simulink model "SimPowACM601"  (R2018b)
settings: Solver=FixedStepAuto  StartTime=0.0  StopTime=Tmu*100  FixedStep=T0  MaxStep=T0  RelTol=1e-3
values from neighbouring files (symbols this model uses):
  add_error = 0    [MathACM601.m]
  ce = 0.0712    [MathACM601.m]
  Cf = 100e-6    (= 0.0001)    [MathACM601.m]
  cm = 0.0712    [MathACM601.m]
  dia = 0.002*Isc*kdt    (= 13.339872)    [MathACM601.m]
  dib = 0.003*Isc*kdt    (= 20.009808)    [MathACM601.m]
  dic = -0.009*Isc*kdt    (= -60.029424)    [MathACM601.m]
  Isc = Udc/R    (= 10.6666666667)    [MathACM601.m]
  J = 0.11e-4    (= 1.1e-05)    [MathACM601.m]
  k = 2    [MathACM601.m]
  KADC = (2^12-1)/3.3    (= 1240.90909091)    [MathACM601.m]
  kda = 1    [MathACM601.m]
  kdb = 0.99    [MathACM601.m]
  kdc = 1.015    [MathACM601.m]
  kdt = Rshunt*Kopa*KADC    (= 625.3065)    [MathACM601.m]
  Ki1 = 1/(Kob*Tt)    (= 375)    [MathACM601.m]
  Ki2 = J*2/(3*8*Tmu^2*ce)    (= 0.514981273408)    [MathACM601.m]
  Kopa = 1.527    [MathACM601.m]
  Kp1 = Te*Ki1    (= 0.5625)    [MathACM601.m]
  Kp2 = 4*Tmu*Ki2    (= 0.0102996254682)    [MathACM601.m]
  Kshunt = 0.001    [MathACM601.m]
  Kv = 1    [MathACM601.m]
  Lsa = Ls    (= 0.002)    [MathACM601.m]
  Lsb = Ls    (= 0.002)    [MathACM601.m]
  Lsc = Ls    (= 0.002)    [MathACM601.m]
  PreMod_3 = 0    [MathACM601.m]
  R = 0.75    [MathACM601.m]
  Ra = R    (= 0.75)    [MathACM601.m]
  Rb = R    (= 0.75)    [MathACM601.m]
  Rc = R    (= 0.75)    [MathACM601.m]
  Rshunt = 0.33    [MathACM601.m]
  Sw = 0    [MathACM601.m]
  T0 = 1e-6    (= 1e-06)    [MathACM601.m]
  tau = 0.00    (= 0)    [MathACM601.m]
  Te = R*Ls    (= 0.0015)    [MathACM601.m]
  Tpwm = 0.5e-4    (= 5e-05)    [MathACM601.m]
  Ts1 = 0.5e-4    (= 5e-05)    [MathACM601.m]
  Ts2 = 0.5e-3    (= 0.0005)    [MathACM601.m]
  Ubias = 1.558    [MathACM601.m]
  Udc = 8    [MathACM601.m]
  zp = 4    [MathACM601.m]
libraries: powerlib x23
settings Model: Creator=ivshu  LastModifiedBy=Шустов Илья
settings SFSimCC: SimUseLocalCustomCode=off
settings RTWCC: RTWUseLocalCustomCode=off
settings CodeAppCC: StateflowObjectComments=on
settings SimscapeCC: SimscapeNormalizeSystem=off

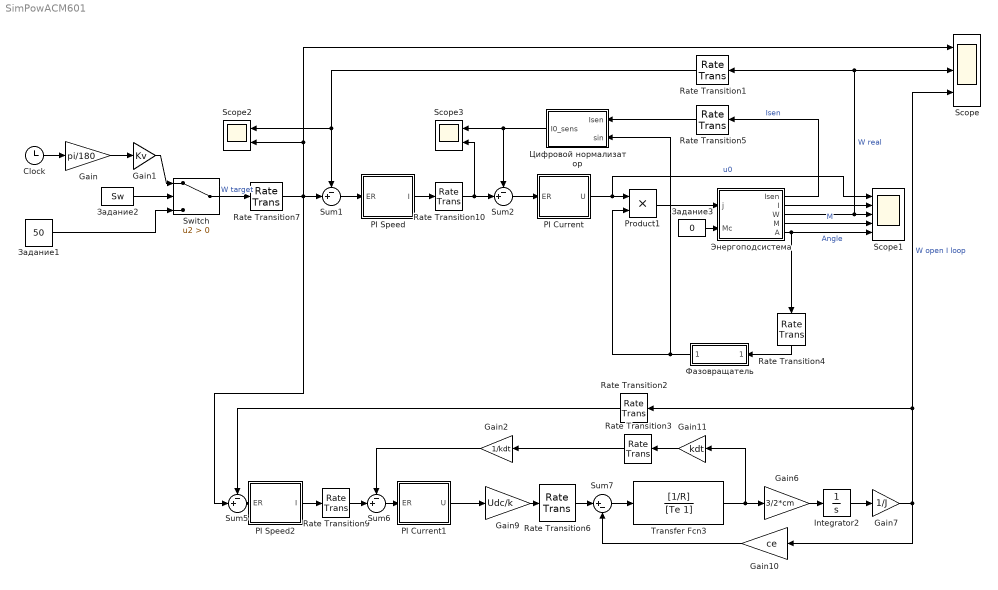
== system SimPowACM601 ==
  Clock : Clock
  Gain : Gain  Gain=pi/180
  Gain1 : Gain  Gain=Kv
  Gain10 : Gain  Gain=ce
  Gain11 : Gain  Gain=kdt
  Gain2 : Gain  Gain=1/kdt
  Gain6 : Gain  Gain=3/2*cm
  Gain7 : Gain  Gain=1/J
  Gain9 : Gain  Gain=Udc/k
  Integrator2 : Integrator
  PI Current : Subsystem
  PI Current1 : Subsystem
  PI Speed : Subsystem
  PI Speed2 : Subsystem
  Product1 : Product
  Rate Transition1 : RateTransition  OutPortSampleTime=Ts2
  Rate Transition{3..5,9..10} (5 alike) : RateTransition  OutPortSampleTime=Ts1
  Rate Transition2 : RateTransition  OutPortSampleTime=Ts2
  Rate Transition6 : RateTransition  OutPortSampleTimeOpt=Inherit
  Rate Transition7 : RateTransition  OutPortSampleTime=Ts2
  Scope : Scope  NumInputPorts=3
  Scope1 : Scope  NumInputPorts=5
  Scope2 : Scope  NumInputPorts=2
  Scope3 : Scope  NumInputPorts=2
  Sum{1..2,5..6} (4 alike) : Sum  Inputs=-+|
  Sum7 : Sum  Inputs=|+-
  Switch : Switch  Criteria=u2 > Threshold
  Transfer Fcn3 : TransferFcn  Numerator=[1/R]  Denominator=[Te 1]
  Задание1 : Constant  Value=50
  Задание2 : Constant  Value=Sw
  Задание3 : Constant  Value=0
  Фазовращатель : Subsystem
  Цифровой нормализатор : Subsystem
  Энергоподсистема : Subsystem
  wires:
  Product1/1 -> Энергоподсистема/1(j)
  Энергоподсистема/3(W) -> Scope1/3, Rate Transition1/1, Scope/2  "W real"
  Sum2/1 -> PI Current/1(ER)
  Цифровой нормализатор/1(I0_sens) -> Sum2/1, Scope3/1
  Rate Transition1/1 -> Sum1/1, Scope2/1
  Задание1/1 -> Switch/3
  Gain/1 -> Gain1/1
  Clock/1 -> Gain/1
  Gain1/1 -> Switch/1
  Энергоподсистема/5(A) -> Rate Transition4/1, Scope1/5  "Angle"
  Энергоподсистема/1(Isen) -> Rate Transition5/1  "Isen"
  Switch/1 -> Rate Transition7/1  "W target"
  Задание2/1 -> Switch/2
  Sum1/1 -> PI Speed/1(ER)
  Sum5/1 -> PI Speed2/1(ER)
  PI Speed2/1(I) -> Rate Transition9/1
  Sum6/1 -> PI Current1/1(ER)
  Transfer Fcn3/1 -> Gain6/1, Gain11/1
  Integrator2/1 -> Gain7/1
  Gain6/1 -> Integrator2/1
  Gain7/1 -> Gain10/1, Rate Transition2/1, Scope/3  "W open I loop"
  Rate Transition2/1 -> Sum5/1
  Rate Transition3/1 -> Gain2/1
  Sum7/1 -> Transfer Fcn3/1
  Rate Transition6/1 -> Sum7/1
  Gain10/1 -> Sum7/2
  Gain11/1 -> Rate Transition3/1
  PI Current/1(U) -> Scope1/1, Product1/1  "u0"
  Rate Transition7/1 -> Sum5/2, Sum1/2, Scope/1, Scope2/2
  Энергоподсистема/4(M) -> Scope1/4  "M"
  Фазовращатель/1(sin(3f)) -> Product1/2, Цифровой нормализатор/2(sin)
  Rate Transition4/1 -> Фазовращатель/1(Angle)
  Rate Transition5/1 -> Цифровой нормализатор/1(Isen)
  Gain9/1 -> Rate Transition6/1
  PI Current1/1(U) -> Gain9/1
  Задание3/1 -> Энергоподсистема/2(Mc)
  Gain2/1 -> Sum6/1
  PI Speed/1(I) -> Rate Transition10/1
  Энергоподсистема/2(I) -> Scope1/2
  Rate Transition9/1 -> Sum6/2
  Rate Transition10/1 -> Scope3/2, Sum2/2

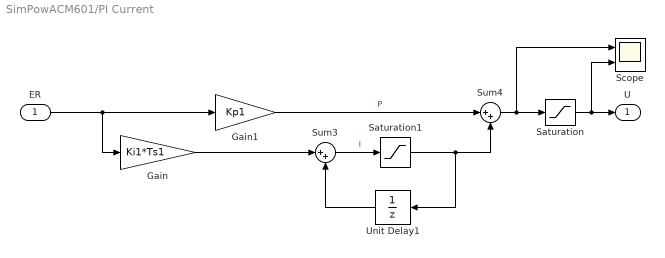
== system SimPowACM601/PI Current ==
  ER : Inport
  Gain : Gain  Gain=Ki1*Ts1
  Gain1 : Gain  Gain=Kp1
  Saturation : Saturate  UpperLimit=1  LowerLimit=-1
  Saturation1 : Saturate  UpperLimit=1  LowerLimit=-1
  Scope : Scope  NumInputPorts=2
  Sum3 : Sum  Inputs=|++
  Sum4 : Sum  Inputs=|++
  Unit Delay1 : UnitDelay  SampleTime=Ts1
  U : Outport
  wires:
  Saturation/1 -> Scope/2, U/1
  Sum4/1 -> Scope/1, Saturation/1
  Gain/1 -> Sum3/1
  Unit Delay1/1 -> Sum3/2
  Sum3/1 -> Saturation1/1  "I"
  Gain1/1 -> Sum4/1  "P"
  ER/1 -> Gain/1, Gain1/1
  Saturation1/1 -> Sum4/2, Unit Delay1/1

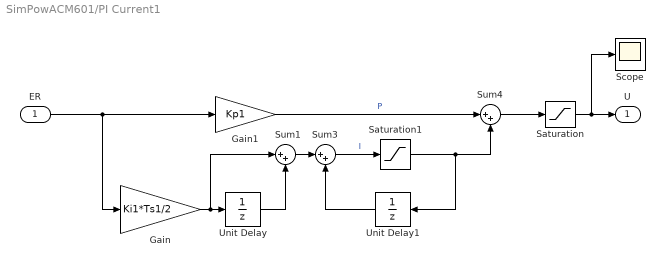
== system SimPowACM601/PI Current1 ==
  ER : Inport
  Gain : Gain  Gain=Ki1*Ts1/2
  Gain1 : Gain  Gain=Kp1
  Saturation : Saturate  UpperLimit=1  LowerLimit=-1
  Saturation1 : Saturate  UpperLimit=1  LowerLimit=-1
  Scope : Scope
  Sum1 : Sum  Inputs=|++
  Sum3 : Sum  Inputs=|++
  Sum4 : Sum  Inputs=|++
  Unit Delay : UnitDelay  SampleTime=Ts1
  Unit Delay1 : UnitDelay  SampleTime=Ts1
  U : Outport
  wires:
  Saturation/1 -> Scope/1, U/1
  Sum4/1 -> Saturation/1
  Gain/1 -> Sum1/1, Unit Delay/1
  Unit Delay/1 -> Sum1/2
  Sum1/1 -> Sum3/1
  Unit Delay1/1 -> Sum3/2
  Sum3/1 -> Saturation1/1  "I"
  Gain1/1 -> Sum4/1  "P"
  ER/1 -> Gain/1, Gain1/1
  Saturation1/1 -> Sum4/2, Unit Delay1/1

== system SimPowACM601/PI Speed ==
  ER : Inport
  Gain : Gain  Gain=Ki2*Ts2
  Gain1 : Gain  Gain=Kp2
  Saturation : Saturate  UpperLimit=Isc  LowerLimit=-Isc
  Saturation1 : Saturate  UpperLimit=Isc  LowerLimit=-Isc
  Scope : Scope  NumInputPorts=2
  Sum3 : Sum  Inputs=|++
  Sum4 : Sum  Inputs=|++
  Unit Delay1 : UnitDelay  SampleTime=Ts2
  I : Outport
  wires:
  Sum4/1 -> Saturation/1
  Gain/1 -> Sum3/1
  Unit Delay1/1 -> Sum3/2
  Sum3/1 -> Saturation1/1  "I"
  Gain1/1 -> Sum4/1  "P"
  ER/1 -> Gain/1, Gain1/1
  Saturation1/1 -> Scope/1, Sum4/2, Unit Delay1/1
  Saturation/1 -> Scope/2, I/1

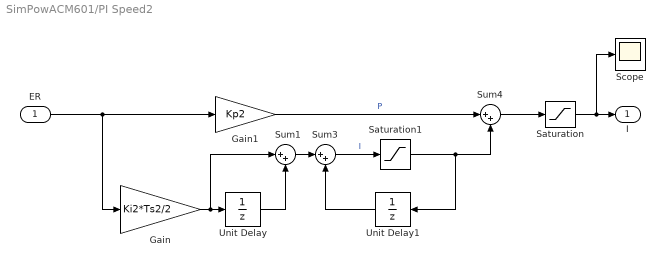
== system SimPowACM601/PI Speed2 ==
  ER : Inport
  Gain : Gain  Gain=Ki2*Ts2/2
  Gain1 : Gain  Gain=Kp2
  Saturation : Saturate  UpperLimit=Isc  LowerLimit=-Isc
  Saturation1 : Saturate  UpperLimit=Isc  LowerLimit=-Isc
  Scope : Scope
  Sum1 : Sum  Inputs=|++
  Sum3 : Sum  Inputs=|++
  Sum4 : Sum  Inputs=|++
  Unit Delay : UnitDelay  SampleTime=Ts2
  Unit Delay1 : UnitDelay  SampleTime=Ts2
  I : Outport
  wires:
  Sum4/1 -> Saturation/1
  Gain/1 -> Sum1/1, Unit Delay/1
  Unit Delay/1 -> Sum1/2
  Sum1/1 -> Sum3/1
  Unit Delay1/1 -> Sum3/2
  Sum3/1 -> Saturation1/1  "I"
  Gain1/1 -> Sum4/1  "P"
  ER/1 -> Gain/1, Gain1/1
  Saturation1/1 -> Sum4/2, Unit Delay1/1
  Saturation/1 -> Scope/1, I/1

== system SimPowACM601/Фазовращатель ==
  Angle : Inport
  Fcn1 : Fcn  Expr=sin(u(1))
  Fcn2 : Fcn  Expr=sin(u(1)+2*pi/3)
  Fcn3 : Fcn  Expr=sin(u(1)-2*pi/3)
  Gain2 : Gain  Gain=zp
  Mux2 : Mux  Inputs=3
  sin(3f) : Outport
  wires:
  Fcn2/1 -> Mux2/2
  Fcn3/1 -> Mux2/3
  Fcn1/1 -> Mux2/1
  Angle/1 -> Gain2/1
  Gain2/1 -> Fcn1/1, Fcn3/1, Fcn2/1
  Mux2/1 -> sin(3f)/1

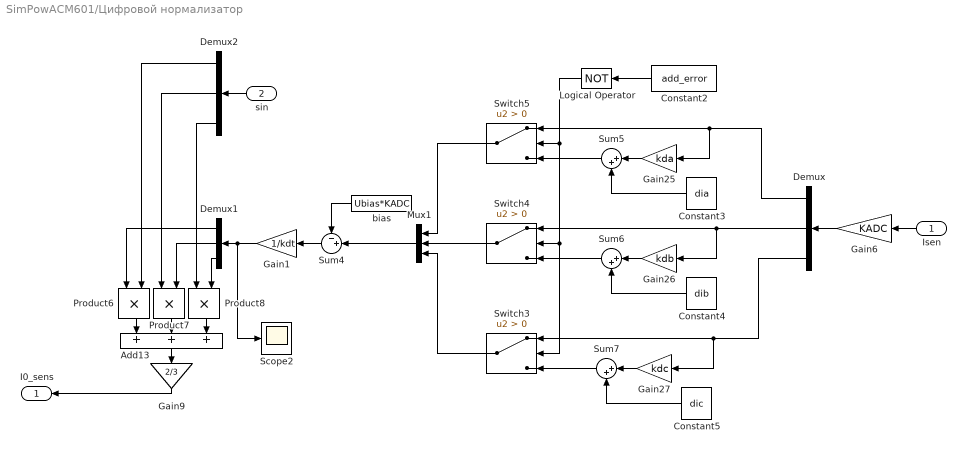
== system SimPowACM601/Цифровой нормализатор ==
  Isen : Inport
  sin : Inport  Port=2
  Add13 : Sum  Inputs=+++
  Constant2 : Constant  Value=add_error
  Constant3 : Constant  Value=dia
  Constant4 : Constant  Value=dib
  Constant5 : Constant  Value=dic
  Demux : Demux  Outputs=3
  Demux1 : Demux  Outputs=3
  Demux2 : Demux  Outputs=3
  Gain1 : Gain  Gain=1/kdt
  Gain25 : Gain  Gain=kda
  Gain26 : Gain  Gain=kdb
  Gain27 : Gain  Gain=kdc
  Gain6 : Gain  Gain=KADC
  Gain9 : Gain  Gain=2/3
  Logical Operator : Logic  Operator=NOT  AllPortsSameDT=off  OutDataTypeStr=boolean
  Mux1 : Mux  Inputs=3
  Product6 : Product
  Product7 : Product
  Product8 : Product
  Scope2 : Scope
  Sum4 : Sum  Inputs=-+|
  Sum5 : Sum  Inputs=|++
  Sum6 : Sum  Inputs=|++
  Sum7 : Sum  Inputs=|++
  Switch3 : Switch  Criteria=u2 > Threshold
  Switch4 : Switch  Criteria=u2 > Threshold
  Switch5 : Switch  Criteria=u2 > Threshold
  bias : Constant  Value=Ubias*KADC
  I0_sens : Outport
  wires:
  Switch4/1 -> Mux1/2
  Switch3/1 -> Mux1/3
  Switch5/1 -> Mux1/1
  Sum5/1 -> Switch5/3
  Constant2/1 -> Logical Operator/1
  Constant3/1 -> Sum5/2
  Gain25/1 -> Sum5/1
  Gain26/1 -> Sum6/1
  Isen/1 -> Gain6/1
  Sum6/1 -> Switch4/3
  Gain27/1 -> Sum7/1
  Sum7/1 -> Switch3/3
  Constant4/1 -> Sum6/2
  Constant5/1 -> Sum7/2
  Logical Operator/1 -> Switch4/2, Switch3/2, Switch5/2
  Demux/3 -> Gain27/1, Switch3/1
  Demux/2 -> Gain26/1, Switch4/1
  Demux/1 -> Gain25/1, Switch5/1
  bias/1 -> Sum4/1
  Sum4/1 -> Gain1/1
  Demux2/3 -> Product8/1
  Demux2/1 -> Product6/2
  Demux1/2 -> Product7/2
  Product6/1 -> Add13/1
  Product7/1 -> Add13/2
  Demux1/1 -> Product6/1
  Product8/1 -> Add13/3
  Gain9/1 -> I0_sens/1
  Add13/1 -> Gain9/1
  Demux1/3 -> Product8/2
  Mux1/1 -> Sum4/2
  Demux2/2 -> Product7/1
  sin/1 -> Demux2/1
  Gain6/1 -> Demux/1
  Gain1/1 -> Scope2/1, Demux1/1

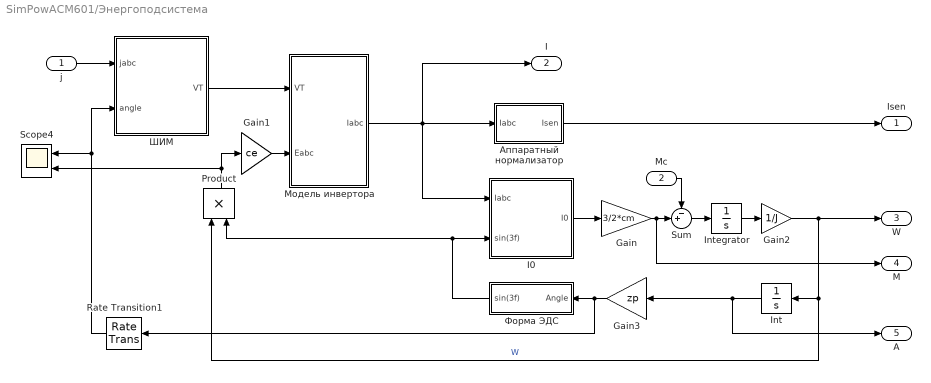
== system SimPowACM601/Энергоподсистема ==
  j : Inport
  Mc : Inport  Port=2
  Gain : Gain  Gain=3/2*cm
  Gain1 : Gain  Gain=ce
  Gain2 : Gain  Gain=1/J
  Gain3 : Gain  Gain=zp
  I0 : Subsystem
  Int : Integrator
  Integrator : Integrator
  Product : Product
  Rate Transition1 : RateTransition  OutPortSampleTime=Ts1
  Scope4 : Scope  NumInputPorts=2
  Sum : Sum  Inputs=-+|
  Аппаратный нормализатор : Subsystem
  Модель инвертора : Subsystem
  Форма ЭДС : Subsystem
  ШИМ : Subsystem
  Isen : Outport
  I : Outport  Port=2
  W : Outport  Port=3
  M : Outport  Port=4
  A : Outport  Port=5
  wires:
  Integrator/1 -> Gain2/1
  Gain2/1 -> Product/1, Int/1, W/1  "W"
  I0/1(I0) -> Gain/1
  Форма ЭДС/1(sin(3f)) -> Product/2, I0/2(sin(3f))
  Sum/1 -> Integrator/1
  Product/1 -> Gain1/1, Scope4/2
  Gain/1 -> M/1, Sum/2
  Модель инвертора/1(Iabc) -> I/1, Аппаратный нормализатор/1(Iabc), I0/1(Iabc)
  Mc/1 -> Sum/1
  Аппаратный нормализатор/1(Isen) -> Isen/1
  Int/1 -> A/1, Gain3/1
  ШИМ/1(VT) -> Модель инвертора/1(" VT")
  j/1 -> ШИМ/1(jabc)
  Gain3/1 -> Rate Transition1/1, Форма ЭДС/1(Angle)
  Gain1/1 -> Модель инвертора/2(" Eabc")
  Rate Transition1/1 -> ШИМ/2(angle), Scope4/1

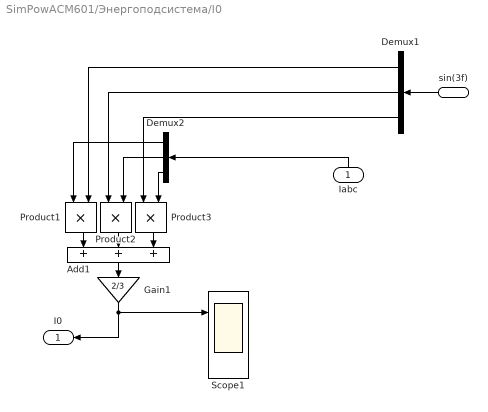
== system SimPowACM601/Энергоподсистема/I0 ==
  Iabc : Inport
  sin(3f) : Inport  Port=2
  Add1 : Sum  Inputs=+++
  Demux1 : Demux  Outputs=3
  Demux2 : Demux  Outputs=3
  Gain1 : Gain  Gain=2/3
  Product1 : Product
  Product2 : Product
  Product3 : Product
  Scope1 : Scope  NumInputPorts=2
  I0 : Outport
  wires:
  sin(3f)/1 -> Demux1/1
  Demux1/3 -> Product3/1
  Demux1/2 -> Product2/1
  Demux1/1 -> Product1/2
  Product3/1 -> Add1/3
  Demux2/1 -> Product1/1
  Add1/1 -> Gain1/1
  Demux2/3 -> Product3/2
  Iabc/1 -> Demux2/1
  Product1/1 -> Add1/1
  Product2/1 -> Add1/2
  Demux2/2 -> Product2/2
  Gain1/1 -> Scope1/1, I0/1

== system SimPowACM601/Энергоподсистема/Аппаратный нормализатор ==
  Iabc : Inport
  Constant1 : Constant  Value=Ubias
  Gain1 : Gain  Gain=Rshunt
  Gain30 : Gain  Gain=Kopa
  Sum1 : Sum  Inputs=++|
  Isen : Outport
  wires:
  Iabc/1 -> Gain1/1
  Constant1/1 -> Sum1/1
  Gain30/1 -> Sum1/2
  Sum1/1 -> Isen/1
  Gain1/1 -> Gain30/1

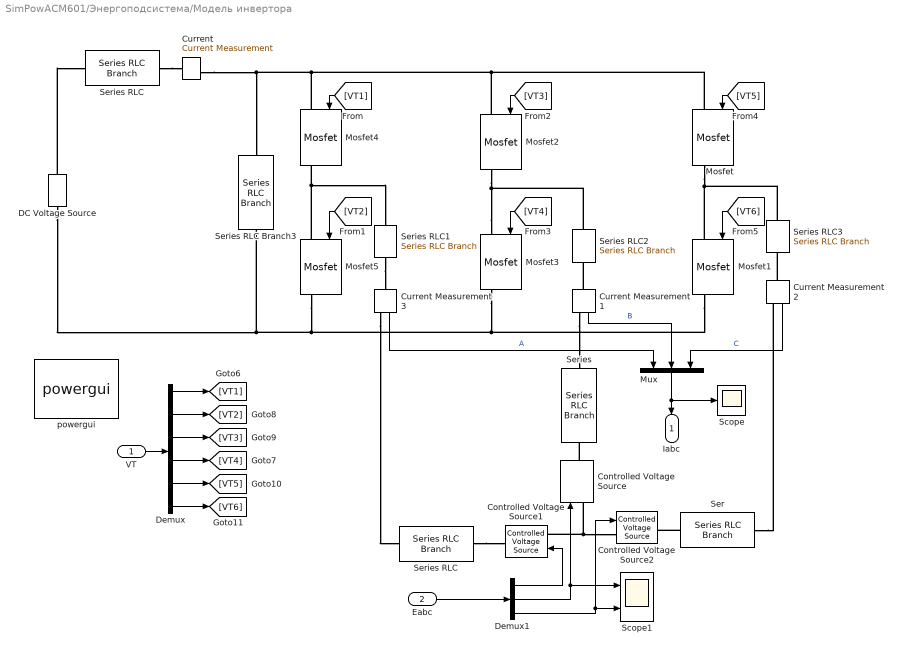
== system SimPowACM601/Энергоподсистема/Модель инвертора ==
  " VT" : Inport
  " Eabc" : Inport  Port=2
  Controlled Voltage Source : powerlib/Electrical Sources/Controlled Voltage Source  Initialize=off  Source_Type=DC  Amplitude=0  Phase=120  Frequency=0  Measurements=None
  Controlled Voltage Source1 : powerlib/Electrical Sources/Controlled Voltage Source  Initialize=off  Source_Type=DC  Amplitude=0  Phase=0  Frequency=0  Measurements=None
  Controlled Voltage Source2 : powerlib/Electrical Sources/Controlled Voltage Source  Initialize=off  Source_Type=DC  Amplitude=0  Phase=240  Frequency=0  Measurements=None
  "Current " : powerlib/Measurements/Current Measurement  PhasorSimulation=off  OutputType=Complex  PSBequivalent=0
  Current Measurement1 : powerlib/Measurements/Current Measurement  PhasorSimulation=off  OutputType=Complex  PSBequivalent=0
  Current Measurement2 : powerlib/Measurements/Current Measurement  PhasorSimulation=off  OutputType=Complex  PSBequivalent=0
  Current Measurement3 : powerlib/Measurements/Current Measurement  PhasorSimulation=off  OutputType=Complex  PSBequivalent=0
  DC Voltage Source : powerlib/Electrical Sources/DC Voltage Source  Amplitude=Udc  Measurements=None
  Demux : Demux  Outputs=6
  Demux1 : Demux  Outputs=3
  Mosfet{,1..5} (6 alike) : powerlib/Power Electronics/Mosfet  Ron=Ron  Lon=0  Rd=0.01  Vfd=Vf  IC=0  Rs=1e5  Cs=inf  Measurements=on
  Mux : Mux  Inputs=3
  Scope : Scope
  Scope1 : Scope  NumInputPorts=2
  Ser : powerlib/Elements/Series RLC Branch  LConnTagsString=__new0  RConnTagsString=__new0  BranchType=RL  Resistance=Rc  Inductance=Lsc  SetiL0=off  InitialCurrent=0  Capacitance=1e-6  Setx0=off  InitialVoltage=0  Measurements=None
  Series : powerlib/Elements/Series RLC Branch  LConnTagsString=__new0  RConnTagsString=__new0  BranchType=RL  Resistance=Rb  Inductance=Lsb  SetiL0=off  InitialCurrent=0  Capacitance=1e-6  Setx0=off  InitialVoltage=0  Measurements=None
  Series RLC : powerlib/Elements/Series RLC Branch  LConnTagsString=__new0  RConnTagsString=__new0  BranchType=RL  Resistance=Ra  Inductance=Lsa  SetiL0=off  InitialCurrent=0  Capacitance=1e-6  Setx0=off  InitialVoltage=0  Measurements=None
  "Series RLC " : powerlib/Elements/Series RLC Branch  LConnTagsString=__new0  RConnTagsString=__new0  BranchType=R  Resistance=0.001  Inductance=1e-3  SetiL0=off  InitialCurrent=0  Capacitance=1e-6  Setx0=off  InitialVoltage=0  Measurements=None
  Series RLC Branch3 : powerlib/Elements/Series RLC Branch  LConnTagsString=__new0  RConnTagsString=__new0  BranchType=C  Resistance=1  Inductance=1e-3  SetiL0=off  InitialCurrent=0  Capacitance=Cf  Setx0=off  InitialVoltage=0  Measurements=None
  Series RLC1 : powerlib/Elements/Series RLC Branch  LConnTagsString=__new0  RConnTagsString=__new0  BranchType=R  Resistance=Rshunt*Kshunt  Inductance=Lsa  SetiL0=off  InitialCurrent=0  Capacitance=1e-6  Setx0=off  InitialVoltage=0  Measurements=None
  Series RLC2 : powerlib/Elements/Series RLC Branch  LConnTagsString=__new0  RConnTagsString=__new0  BranchType=R  Resistance=Rshunt*Kshunt  Inductance=Lsa  SetiL0=off  InitialCurrent=0  Capacitance=1e-6  Setx0=off  InitialVoltage=0  Measurements=None
  Series RLC3 : powerlib/Elements/Series RLC Branch  LConnTagsString=__new0  RConnTagsString=__new0  BranchType=R  Resistance=Rshunt*Kshunt  Inductance=Lsa  SetiL0=off  InitialCurrent=0  Capacitance=1e-6  Setx0=off  InitialVoltage=0  Measurements=None
  powergui : powerlib/powergui  Priority=1  SimulationMode=Discrete  SampleTime=T0  frequency=60  Iterations=50  frequencyindice=0  Pbase=100e6  ErrMax=1e-4  UnitsV=kV  UnitsW=MW  buscounter=0  FunctionMessages=off  echomessages=off  EnableUseOfTLC=off  CurrentSourceSwitches=off  DisableSnubberDevices=off  DisableRonSwitches=off  DisableVfSwitches=off  DisplayEquations=off  SolverType=Tustin/Backward Euler (TBE)  Interpol=off  ExternalGateDelay=off  methode=off  Ts=100  x0status=blocks  SPID=off  SwTol=0  HookPort=off  RestoreLinks=warning  ResistiveCurrentMeasurement=off  Frange=[0:2:500]  Ylog=off  Xlog=on  ShowGrid=off  save=off  variable=ZData  structure=0  ZoomFFT=off  StartTime=0.0  cycles=1  DisplayStyle=1  fundamental=60  FreqAxis=off  MaxFrequency=1000  frequencyindicesteady=1  RmsSteady=1  display=off
  Iabc : Outport
  wires:
  " VT"/1 -> Demux/1
  Mux/1 -> Scope/1, Iabc/1
  Current Measurement3/1 -> Mux/1  "A"
  [VT1] -> Mosfet4/1
  Demux/4 -> [VT4]
  Demux/6 -> [VT6]
  Current Measurement2/1 -> Mux/3  "C"
  Current Measurement1/1 -> Mux/2  "B"
  [VT6] -> Mosfet1/1
  [VT5] -> Mosfet/1
  Demux/3 -> [VT3]
  Demux/2 -> [VT2]
  Demux/5 -> [VT5]
  Demux/1 -> [VT1]
  [VT3] -> Mosfet2/1
  [VT2] -> Mosfet5/1
  [VT4] -> Mosfet3/1
  Demux1/1 -> Controlled Voltage Source1/1
  Demux1/2 -> Scope1/1, Controlled Voltage Source/1
  Demux1/3 -> Scope1/2, Controlled Voltage Source2/1
  " Eabc"/1 -> Demux1/1
  connections:
  Ser/LConn1 -- Current Measurement2/RConn1
  Mosfet3/LConn1 -- Series RLC2/LConn1 -- Mosfet2/RConn1
  Series RLC Branch3/RConn1 -- DC Voltage Source/LConn1 -- Mosfet5/RConn1 -- Mosfet3/RConn1 -- Mosfet1/RConn1
  Series RLC1/RConn1 -- Current Measurement3/LConn1
  Mosfet1/LConn1 -- Series RLC3/LConn1 -- Mosfet/RConn1
  DC Voltage Source/RConn1 -- "Series RLC "/LConn1
  "Current "/RConn1 -- Series RLC Branch3/LConn1 -- Mosfet2/LConn1 -- Mosfet/LConn1 -- Mosfet4/LConn1
  Controlled Voltage Source/LConn1 -- Controlled Voltage Source1/LConn1 -- Controlled Voltage Source2/LConn1
  Controlled Voltage Source/RConn1 -- Series/RConn1
  Current Measurement3/RConn1 -- Series RLC/LConn1
  Ser/RConn1 -- Controlled Voltage Source2/RConn1
  Series RLC/RConn1 -- Controlled Voltage Source1/RConn1
  Current Measurement1/RConn1 -- Series/LConn1
  "Series RLC "/RConn1 -- "Current "/LConn1
  Mosfet5/LConn1 -- Mosfet4/RConn1 -- Series RLC1/LConn1
  Current Measurement1/LConn1 -- Series RLC2/RConn1
  Current Measurement2/LConn1 -- Series RLC3/RConn1

== system SimPowACM601/Энергоподсистема/Форма ЭДС ==
  Angle : Inport
  Fcn1 : Fcn  Expr=sin(u(1))
  Fcn2 : Fcn  Expr=sin(u(1)+2*pi/3)
  Fcn3 : Fcn  Expr=sin(u(1)-2*pi/3)
  Mux2 : Mux  Inputs=3
  sin(3f) : Outport
  wires:
  Fcn2/1 -> Mux2/2
  Fcn3/1 -> Mux2/3
  Fcn1/1 -> Mux2/1
  Mux2/1 -> sin(3f)/1
  Angle/1 -> Fcn2/1, Fcn1/1, Fcn3/1

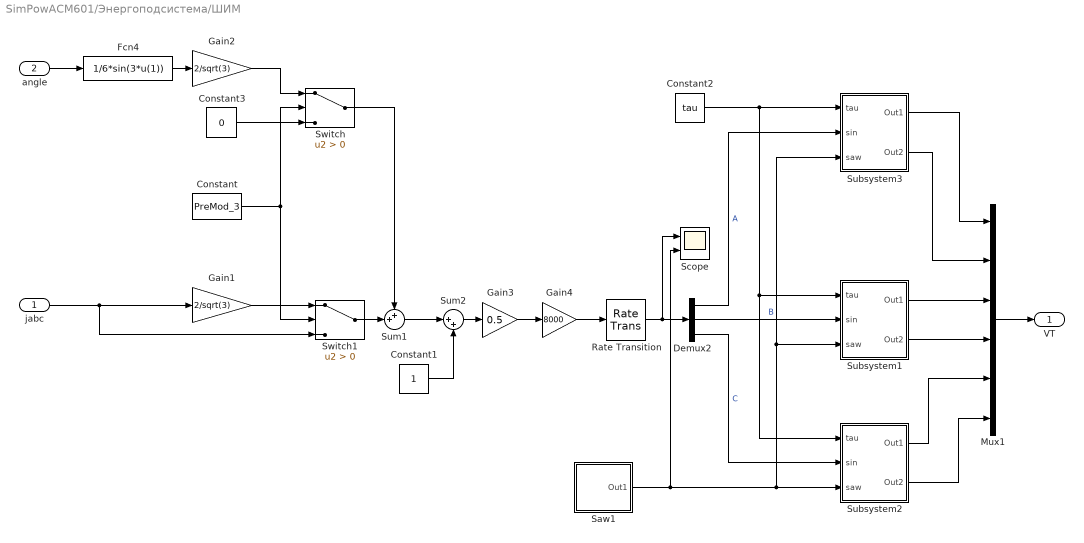
== system SimPowACM601/Энергоподсистема/ШИМ ==
  jabc : Inport
  angle : Inport  Port=2
  Constant : Constant  Value=PreMod_3
  Constant1 : Constant
  Constant2 : Constant  Value=tau
  Constant3 : Constant  Value=0
  Demux2 : Demux  Outputs=3
  Fcn4 : Fcn  Expr=1/6*sin(3*u(1))
  Gain1 : Gain  Gain=2/sqrt(3)
  Gain2 : Gain  Gain=2/sqrt(3)
  Gain3 : Gain  Gain=0.5
  Gain4 : Gain  Gain=8000
  Mux1 : Mux  Inputs=6
  Rate Transition : RateTransition  OutPortSampleTimeOpt=Inherit  OutPortSampleTime=-
  Saw1 : Subsystem
  Scope : Scope  NumInputPorts=2
  Subsystem1 : Subsystem
  Subsystem2 : Subsystem
  Subsystem3 : Subsystem
  Sum1 : Sum  Inputs=++|
  Sum2 : Sum  Inputs=|++
  Switch : Switch  Criteria=u2 > Threshold
  Switch1 : Switch  Criteria=u2 > Threshold
  VT : Outport
  wires:
  Saw1/1(Out1) -> Scope/2, Subsystem1/3(saw), Subsystem3/3(saw), Subsystem2/3(saw)
  Demux2/2 -> Subsystem1/2(sin)  "B"
  Subsystem1/1(Out1) -> Mux1/3
  Subsystem1/2(Out2) -> Mux1/4
  Demux2/3 -> Subsystem2/2(sin)  "C"
  Constant2/1 -> Subsystem3/1(tau), Subsystem2/1(tau), Subsystem1/1(tau)
  Demux2/1 -> Subsystem3/2(sin)  "A"
  Subsystem3/1(Out1) -> Mux1/1
  Subsystem3/2(Out2) -> Mux1/2
  Sum1/1 -> Sum2/1
  Gain2/1 -> Switch/1
  Constant/1 -> Switch/2, Switch1/2
  jabc/1 -> Gain1/1, Switch1/3
  Constant3/1 -> Switch/3
  Fcn4/1 -> Gain2/1
  Switch1/1 -> Sum1/2
  Switch/1 -> Sum1/1
  angle/1 -> Fcn4/1
  Gain1/1 -> Switch1/1
  Constant1/1 -> Sum2/2
  Sum2/1 -> Gain3/1
  Gain3/1 -> Gain4/1
  Gain4/1 -> Rate Transition/1
  Subsystem2/2(Out2) -> Mux1/6
  Subsystem2/1(Out1) -> Mux1/5
  Rate Transition/1 -> Scope/1, Demux2/1
  Mux1/1 -> VT/1

== system SimPowACM601/Энергоподсистема/ШИМ/Saw1 ==
  Constant2 : Constant
  Gain1 : Gain  Gain=8000
  Gain3 : Gain  Gain=2/Tpwm
  Integrator : Integrator
  Pulse Generator : DiscretePulseGenerator  PulseType=Time based  Amplitude=2  Period=Tpwm  PulseWidth=50
  Scope : Scope  NumInputPorts=4
  Sum9 : Sum  Inputs=|+-
  Out1 : Outport
  wires:
  Gain1/1 -> Scope/3, Integrator/1
  Gain3/1 -> Gain1/1
  Sum9/1 -> Scope/2, Gain3/1
  Pulse Generator/1 -> Scope/1, Sum9/1
  Constant2/1 -> Sum9/2
  Integrator/1 -> Out1/1, Scope/4

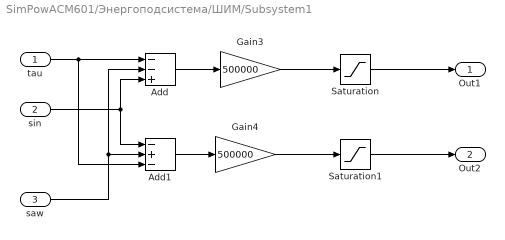
== system SimPowACM601/Энергоподсистема/ШИМ/Subsystem1 ==
  tau : Inport
  sin : Inport  Port=2
  saw : Inport  Port=3
  Add : Sum  Inputs=--+
  Add1 : Sum  Inputs=-+-
  Gain3 : Gain  Gain=500000
  Gain4 : Gain  Gain=500000
  Saturation : Saturate  UpperLimit=10  LowerLimit=0
  Saturation1 : Saturate  UpperLimit=10  LowerLimit=0
  Out1 : Outport
  Out2 : Outport  Port=2
  wires:
  Add/1 -> Gain3/1
  saw/1 -> Add/2, Add1/2
  Gain4/1 -> Saturation1/1
  Gain3/1 -> Saturation/1
  sin/1 -> Add/3, Add1/1
  Add1/1 -> Gain4/1
  tau/1 -> Add1/3, Add/1
  Saturation1/1 -> Out2/1
  Saturation/1 -> Out1/1

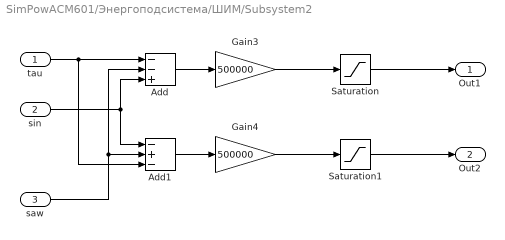
== system SimPowACM601/Энергоподсистема/ШИМ/Subsystem2 ==
  tau : Inport
  sin : Inport  Port=2
  saw : Inport  Port=3
  Add : Sum  Inputs=--+
  Add1 : Sum  Inputs=-+-
  Gain3 : Gain  Gain=500000
  Gain4 : Gain  Gain=500000
  Saturation : Saturate  UpperLimit=10  LowerLimit=0
  Saturation1 : Saturate  UpperLimit=10  LowerLimit=0
  Out1 : Outport
  Out2 : Outport  Port=2
  wires:
  Add/1 -> Gain3/1
  saw/1 -> Add/2, Add1/2
  Gain4/1 -> Saturation1/1
  Gain3/1 -> Saturation/1
  sin/1 -> Add/3, Add1/1
  Add1/1 -> Gain4/1
  tau/1 -> Add1/3, Add/1
  Saturation1/1 -> Out2/1
  Saturation/1 -> Out1/1

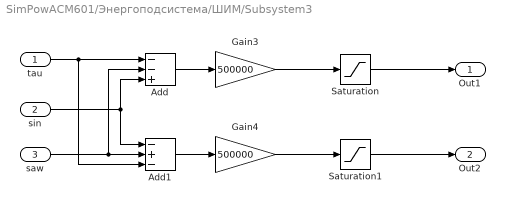
== system SimPowACM601/Энергоподсистема/ШИМ/Subsystem3 ==
  tau : Inport
  sin : Inport  Port=2
  saw : Inport  Port=3
  Add : Sum  Inputs=--+
  Add1 : Sum  Inputs=-+-
  Gain3 : Gain  Gain=500000
  Gain4 : Gain  Gain=500000
  Saturation : Saturate  UpperLimit=10  LowerLimit=0
  Saturation1 : Saturate  UpperLimit=10  LowerLimit=0
  Out1 : Outport
  Out2 : Outport  Port=2
  wires:
  Add/1 -> Gain3/1
  saw/1 -> Add/2, Add1/2
  Gain4/1 -> Saturation1/1
  Gain3/1 -> Saturation/1
  sin/1 -> Add/3, Add1/1
  Add1/1 -> Gain4/1
  tau/1 -> Add1/3, Add/1
  Saturation1/1 -> Out2/1
  Saturation/1 -> Out1/1
